simulink model "L1"  (R2023b)
settings: Solver=VariableStepAuto  StartTime=0.0  StopTime=10.0  RelTol=1e-3
values from neighbouring files (symbols this model uses):
  gravity = Airplane_data(52)    [Data_edit.m]
libraries: vrlib x6, dspmathops x4, matrix_library x1
settings Model: Creator=saifg  LastModifiedBy=saifg

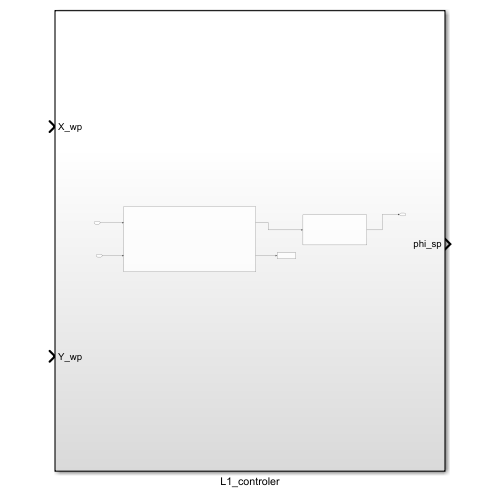
[thumbnail: Simulink's stored preview of the top-level diagram]
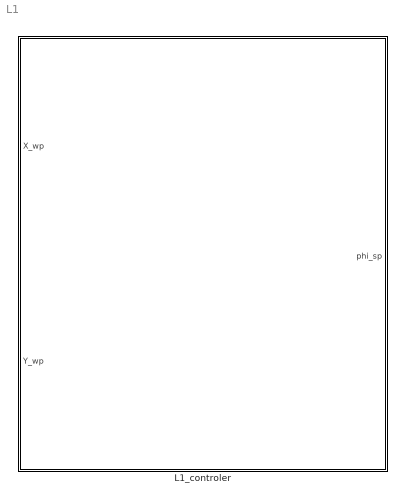
== system L1 ==
  L1_controler : Subsystem

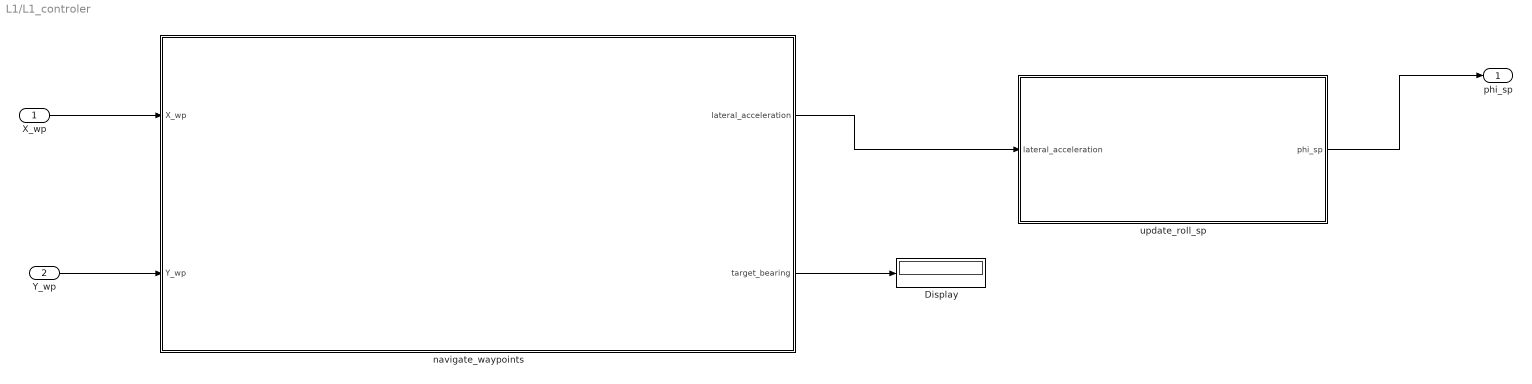
== system L1/L1_controler ==
  X_wp : Inport
  Y_wp : Inport  Port=2
  Display : Display
  navigate_waypoints : Subsystem
  update_roll_sp : Subsystem
  phi_sp : Outport
  wires:
  X_wp/1 -> navigate_waypoints/1(X_wp)
  Y_wp/1 -> navigate_waypoints/2(Y_wp)
  navigate_waypoints/2(target_bearing) -> Display/1
  navigate_waypoints/1(lateral_acceleration) -> update_roll_sp/1(lateral_acceleration)
  update_roll_sp/1(phi_sp) -> phi_sp/1

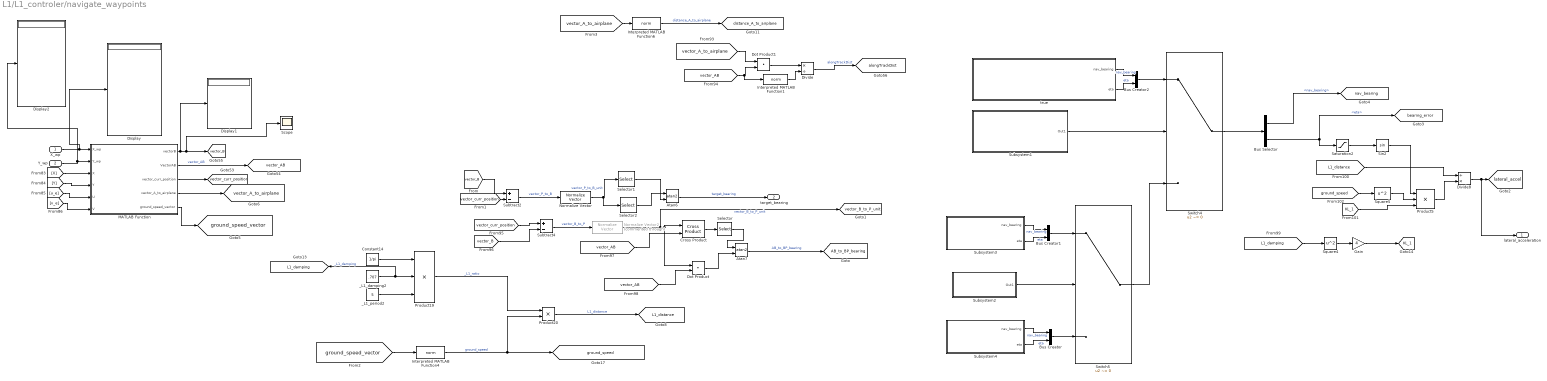
== system L1/L1_controler/navigate_waypoints ==
  X_wp : Inport
  Y_wp : Inport  Port=2
  Atan6 : Trigonometry  Operator=atan2
  Atan7 : Trigonometry  Operator=atan2
  Bus Creator : BusCreator  Inputs=2
  Bus Creator1 : BusCreator  Inputs=2
  Bus Creator2 : BusCreator  Inputs=2
  Bus Selector : BusSelector  OutputSignals=nav_bearing,eta
  Constant14 : Constant  Value=1/pi
  Cross Product : matrix_library/Cross Product
  Display : Display
  Display1 : Display
  Display2 : Display
  Divide : Product  Inputs=*/
  Divide8 : Product  Inputs=/*
  Dot Product : DotProduct  OutDataTypeStr=Inherit: Inherit via internal rule
  Dot Product1 : DotProduct  OutDataTypeStr=Inherit: Inherit via internal rule
  Gain : Gain  Gain=4
  Interpreted MATLAB Function1 : MATLABFcn  MATLABFcn=norm
  Interpreted MATLAB Function4 : MATLABFcn  MATLABFcn=norm
  Interpreted MATLAB Function6 : MATLABFcn  MATLABFcn=norm
  MATLAB Function : MATLAB Function  TreatAsAtomicUnit=on
  Normalize Vector : vrlib/Utilities/Normalize Vector  maxzero=0
  Normalize Vector2 : vrlib/Utilities/Normalize Vector  Commented=through  maxzero=0
  Product19 : Product  Inputs=3
  Product20 : Product
  Product5 : Product  Inputs=3
  Saturation2 : Saturate  UpperLimit=pi/2  LowerLimit=-pi/2
  Scope : Scope
  Selector : Selector  InputPortWidth=3  IndexOptions=Index vector (dialog)  Indices=3  OutputSizes=1
  Selector1 : Selector  InputPortWidth=3  IndexOptions=Index vector (dialog)  Indices=1  OutputSizes=1
  Selector2 : Selector  InputPortWidth=3  IndexOptions=Index vector (dialog)  Indices=2  OutputSizes=1
  Sin2 : Trigonometry
  Square4 : Math  Operator=square
  Square5 : Math  Operator=square
  Subsystem1 : Subsystem
  Subsystem2 : Subsystem
  Subsystem3 : Subsystem
  Subsystem4 : Subsystem
  Subtract2 : Sum  Inputs=+-
  Subtract4 : Sum  Inputs=+-
  Switch4 : Switch  Criteria=u2 ~= 0  SaturateOnIntegerOverflow=off  InputSameDT=off
  Switch5 : Switch  Criteria=u2 ~= 0  SaturateOnIntegerOverflow=off  InputSameDT=off
  _L1_damping2 : Constant  Value=.707
  _L1_period2 : Constant  Value=5
  true : Subsystem
  lateral_acceleration : Outport
  target_bearing : Outport  Port=2
  tag scope: AB_to_BP_bearing=global, KL_1=global, L1_damping=global, L1_distance=global, alongTrackDist=global, bearing_error=global, distance_A_to_airplane=global, ground_speed=global, ground_speed_vector=global, lateral_accel=global, nav_bearing=global, vector_AB=global, vector_A_to_airplane=global, vector_B=global, vector_B_to_P_unit=global, vector_curr_position=global
  wires:
  Dot Product/1 -> Atan7/2
  Divide/1 -> [alongTrackDist]  "alongTrackDist"
  Product19/1 -> Product20/1  "_L1_ratio"
  [ground_speed] -> Square5/1
  Sin2/1 -> Product5/1
  Interpreted MATLAB Function4/1 -> Product20/2, [ground_speed]  "ground_speed"
  MATLAB Function/2(VectorAB) -> [vector_AB]  "vector_AB"
  Normalize Vector/1 -> Selector2/1, Selector1/1  "vector_P_to_B_unit"
  Product20/1 -> [L1_distance]  "L1_distance"
  Y_wp/1 -> Display2/1, MATLAB Function/2(Y_wp)
  Atan7/1 -> [AB_to_BP_bearing]  "AB_to_BP_bearing"
  [L1_damping] -> Square4/1
  Constant14/1 -> Product19/1
  Subsystem1/1(Out1) -> Switch4/2
  Subtract2/1 -> Normalize Vector/1  "vector_P_to_B"
  [vector_A_to_airplane] -> Dot Product1/1
  X_wp/1 -> MATLAB Function/1(X_wp), Display/1
  [X] -> MATLAB Function/3(X)
  Divide8/1 -> lateral_acceleration/1, [lateral_accel]
  [Y] -> MATLAB Function/4(Y)
  Normalize Vector2/1 -> Dot Product/1, Cross Product/1, [vector_B_to_P_unit]  "vector_B_to_P_unit"
  Bus Creator2/1 -> Switch4/1
  [vector_B] -> Subtract4/2
  Subtract4/1 -> Normalize Vector2/1  "vector_B_to_P"
  [vector_curr_position] -> Subtract4/1
  [vector_AB] -> Interpreted MATLAB Function1/1, Dot Product1/2
  _L1_period2/1 -> Product19/3
  Bus Selector/1 -> [nav_bearing]  "<nav_bearing>"
  true/2(eta) -> Bus Creator2/2  "eta"
  _L1_damping2/1 -> [L1_damping], Product19/2  "_L1_damping"
  Bus Selector/2 -> Saturation2/1, [bearing_error]  "<eta>"
  Interpreted MATLAB Function6/1 -> [distance_A_to_airplane]  "distance_A_to_airplane"
  Switch5/1 -> Switch4/3
  Switch4/1 -> Bus Selector/1
  true/1(nav_bearing) -> Bus Creator2/1  "nav_bearing"
  Square4/1 -> Gain/1
  [L1_distance] -> Divide8/1
  Subsystem4/1(nav_bearing) -> Bus Creator/1  "nav_bearing"
  Subsystem4/2(eta) -> Bus Creator/2  "eta"
  Subsystem3/1(nav_bearing) -> Bus Creator1/1  "nav_bearing"
  Subsystem3/2(eta) -> Bus Creator1/2  "eta"
  Subsystem2/1(Out1) -> Switch5/2
  Saturation2/1 -> Sin2/1
  Product5/1 -> Divide8/2
  Atan6/1 -> target_bearing/1  "target_bearing"
  Gain/1 -> [KL_1]
  Square5/1 -> Product5/2
  [KL_1] -> Product5/3
  Bus Creator/1 -> Switch5/3
  Bus Creator1/1 -> Switch5/1
  [vector_AB] -> Dot Product/2
  Selector/1 -> Atan7/1
  Dot Product1/1 -> Divide/1
  Interpreted MATLAB Function1/1 -> Divide/2
  [vector_B] -> Subtract2/1
  [vector_curr_position] -> Subtract2/2
  MATLAB Function/1(vectorB) -> Display1/1, Scope/1, [vector_B]
  [vector_AB] -> Cross Product/2
  [u_e] -> MATLAB Function/5(U)
  [v_e] -> MATLAB Function/6(V)
  MATLAB Function/5(ground_speed_vector) -> [ground_speed_vector]
  [ground_speed_vector] -> Interpreted MATLAB Function4/1
  MATLAB Function/3(vector_curr_position) -> [vector_curr_position]
  MATLAB Function/4(vector_A_to_airplane) -> [vector_A_to_airplane]
  [vector_A_to_airplane] -> Interpreted MATLAB Function6/1
  Selector2/1 -> Atan6/1
  Selector1/1 -> Atan6/2
  Cross Product/1 -> Selector/1

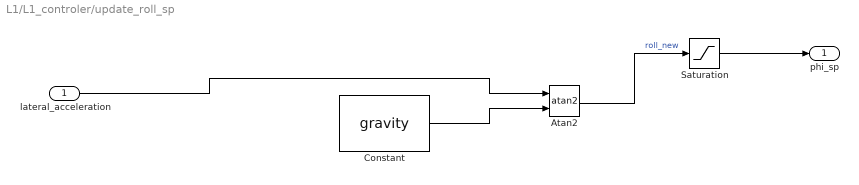
== system L1/L1_controler/update_roll_sp ==
  lateral_acceleration : Inport
  Atan2 : Trigonometry  Operator=atan2
  Constant : Constant  Value=gravity
  Saturation : Saturate  UpperLimit=deg2rad(70)  LowerLimit=-deg2rad(70)
  phi_sp : Outport
  wires:
  Saturation/1 -> phi_sp/1
  Constant/1 -> Atan2/2
  Atan2/1 -> Saturation/1  "roll_new"
  lateral_acceleration/1 -> Atan2/1

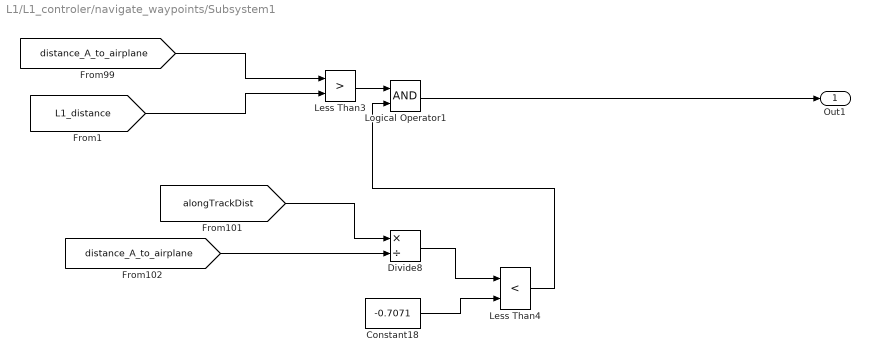
== system L1/L1_controler/navigate_waypoints/Subsystem1 ==
  Constant18 : Constant  Value=-0.7071
  Divide8 : Product  Inputs=*/
  Less Than3 : RelationalOperator  Operator=>  OutDataTypeStr=boolean  RndMeth=Simplest  InputSameDT=off
  Less Than4 : RelationalOperator  Operator=<  OutDataTypeStr=boolean  RndMeth=Simplest  InputSameDT=off
  Logical Operator1 : Logic  AllPortsSameDT=off  OutDataTypeStr=boolean
  Out1 : Outport
  wires:
  Less Than3/1 -> Logical Operator1/1
  Less Than4/1 -> Logical Operator1/2
  [distance_A_to_airplane] -> Less Than3/1
  Divide8/1 -> Less Than4/1
  Constant18/1 -> Less Than4/2
  [alongTrackDist] -> Divide8/1
  [L1_distance] -> Less Than3/2
  [distance_A_to_airplane] -> Divide8/2
  Logical Operator1/1 -> Out1/1

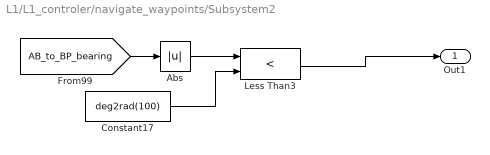
== system L1/L1_controler/navigate_waypoints/Subsystem2 ==
  Abs : Abs  SaturateOnIntegerOverflow=off
  Constant17 : Constant  Value=deg2rad(100)
  Less Than3 : RelationalOperator  Operator=<  OutDataTypeStr=boolean  RndMeth=Simplest  InputSameDT=off
  Out1 : Outport
  wires:
  Constant17/1 -> Less Than3/2
  [AB_to_BP_bearing] -> Abs/1
  Abs/1 -> Less Than3/1
  Less Than3/1 -> Out1/1

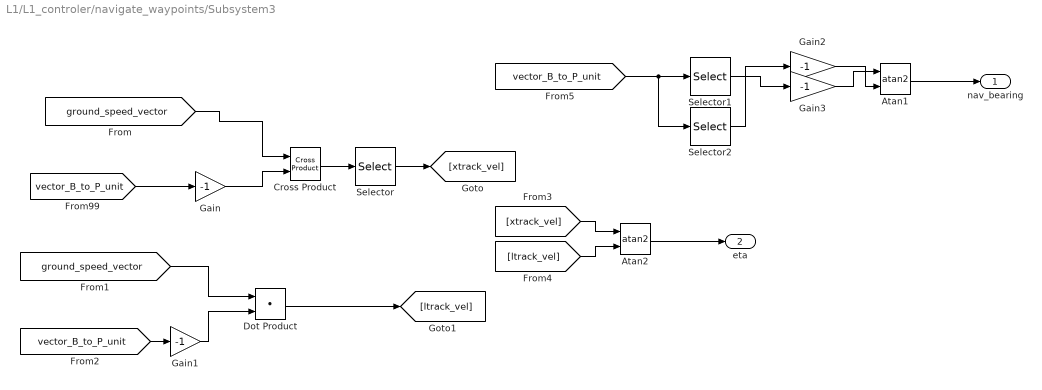
== system L1/L1_controler/navigate_waypoints/Subsystem3 ==
  Atan1 : Trigonometry  Operator=atan2
  Atan2 : Trigonometry  Operator=atan2
  Cross Product : vrlib/Utilities/Cross Product
  Dot Product : DotProduct  OutDataTypeStr=Inherit: Inherit via internal rule
  Gain{,1..3} (4 alike) : Gain  Gain=-1
  Selector : Selector  InputPortWidth=3  IndexOptions=Index vector (dialog)  Indices=3  OutputSizes=1
  Selector1 : Selector  InputPortWidth=3  IndexOptions=Index vector (dialog)  Indices=1  OutputSizes=1
  Selector2 : Selector  InputPortWidth=3  IndexOptions=Index vector (dialog)  Indices=2  OutputSizes=1
  nav_bearing : Outport
  eta : Outport  Port=2
  wires:
  [vector_B_to_P_unit] -> Gain/1
  Dot Product/1 -> [ltrack_vel]
  Gain1/1 -> Dot Product/2
  [vector_B_to_P_unit] -> Gain1/1
  [ground_speed_vector] -> Dot Product/1
  [xtrack_vel] -> Atan2/1
  [ltrack_vel] -> Atan2/2
  Atan2/1 -> eta/1
  Gain3/1 -> Atan1/1
  Gain2/1 -> Atan1/2
  Atan1/1 -> nav_bearing/1
  Gain/1 -> Cross Product/2
  [ground_speed_vector] -> Cross Product/1
  Cross Product/1 -> Selector/1
  Selector/1 -> [xtrack_vel]
  [vector_B_to_P_unit] -> Selector2/1, Selector1/1
  Selector1/1 -> Gain3/1
  Selector2/1 -> Gain2/1

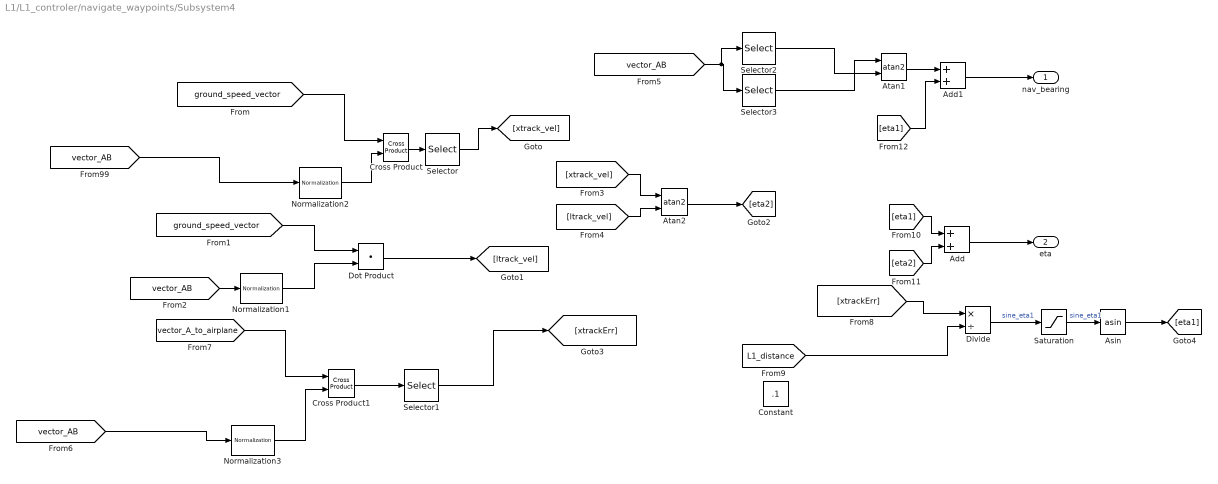
== system L1/L1_controler/navigate_waypoints/Subsystem4 ==
  Add : Sum
  Add1 : Sum
  Asin : Trigonometry  Operator=asin
  Atan1 : Trigonometry  Operator=atan2
  Atan2 : Trigonometry  Operator=atan2
  Constant : Constant  Value=.1
  Cross Product : vrlib/Utilities/Cross Product
  Cross Product1 : vrlib/Utilities/Cross Product
  Divide : Product  Inputs=*/
  Dot Product : DotProduct  OutDataTypeStr=Inherit: Inherit via internal rule
  Normalization1 : dspmathops/Normalization  NormType=2-norm  Bias=1e-10  NormOver=Each column  Dimension=1  roundingMode=Floor  overflowMode=off  accumDataTypeStr=Inherit: Same as product output  accumLastDataTypeStr=Inherit: Same as product output  outputDataTypeStr=Inherit: Same as product output  outputMin=[]  outputMax=[]  outputLastDataTypeStr=Inherit: Same as product output
  Normalization2 : dspmathops/Normalization  NormType=2-norm  Bias=1e-10  NormOver=Each column  Dimension=1  roundingMode=Floor  overflowMode=off  accumDataTypeStr=Inherit: Same as product output  accumLastDataTypeStr=Inherit: Same as product output  outputDataTypeStr=Inherit: Same as product output  outputMin=[]  outputMax=[]  outputLastDataTypeStr=Inherit: Same as product output
  Normalization3 : dspmathops/Normalization  NormType=2-norm  Bias=1e-10  NormOver=Each column  Dimension=1  roundingMode=Floor  overflowMode=off  accumDataTypeStr=Inherit: Same as product output  accumLastDataTypeStr=Inherit: Same as product output  outputDataTypeStr=Inherit: Same as product output  outputMin=[]  outputMax=[]  outputLastDataTypeStr=Inherit: Same as product output
  Saturation : Saturate  UpperLimit=sin(pi/4)  LowerLimit=-sin(pi/4)
  Selector : Selector  InputPortWidth=3  IndexOptions=Index vector (dialog)  Indices=[3]  OutputSizes=1
  Selector1 : Selector  InputPortWidth=3  IndexOptions=Index vector (dialog)  Indices=[3]  OutputSizes=1
  Selector2 : Selector  InputPortWidth=3  IndexOptions=Index vector (dialog)  Indices=1  OutputSizes=1
  Selector3 : Selector  InputPortWidth=3  IndexOptions=Index vector (dialog)  Indices=2  OutputSizes=1
  nav_bearing : Outport
  eta : Outport  Port=2
  wires:
  [ltrack_vel] -> Atan2/2
  [xtrack_vel] -> Atan2/1
  [ground_speed_vector] -> Dot Product/1
  [vector_AB] -> Normalization1/1
  Dot Product/1 -> [ltrack_vel]
  Atan2/1 -> [eta2]
  [xtrackErr] -> Divide/1
  [L1_distance] -> Divide/2
  Divide/1 -> Saturation/1  "sine_eta1"
  Saturation/1 -> Asin/1  "sine_eta1"
  Asin/1 -> [eta1]
  [eta1] -> Add/1
  [eta2] -> Add/2
  Add/1 -> eta/1
  Atan1/1 -> Add1/1
  [eta1] -> Add1/2
  Add1/1 -> nav_bearing/1
  [vector_AB] -> Normalization2/1
  [ground_speed_vector] -> Cross Product/1
  Cross Product/1 -> Selector/1
  Selector/1 -> [xtrack_vel]
  [vector_A_to_airplane] -> Cross Product1/1
  [vector_AB] -> Normalization3/1
  Cross Product1/1 -> Selector1/1
  Selector1/1 -> [xtrackErr]
  Normalization1/1 -> Dot Product/2
  Normalization2/1 -> Cross Product/2
  Normalization3/1 -> Cross Product1/2
  [vector_AB] -> Selector2/1, Selector3/1
  Selector3/1 -> Atan1/1
  Selector2/1 -> Atan1/2

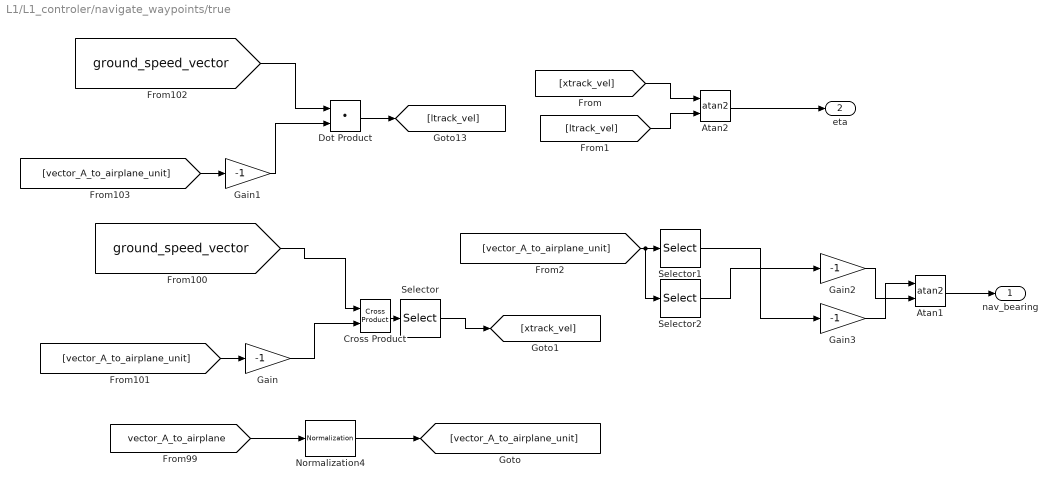
== system L1/L1_controler/navigate_waypoints/true ==
  Atan1 : Trigonometry  Operator=atan2
  Atan2 : Trigonometry  Operator=atan2
  Cross Product : vrlib/Utilities/Cross Product
  Dot Product : DotProduct  OutDataTypeStr=Inherit: Inherit via internal rule
  Gain{,1..3} (4 alike) : Gain  Gain=-1
  Normalization4 : dspmathops/Normalization  NormType=2-norm  Bias=1e-10  NormOver=Each column  Dimension=1  roundingMode=Floor  overflowMode=off  accumDataTypeStr=Inherit: Same as product output  accumLastDataTypeStr=Inherit: Same as product output  outputDataTypeStr=Inherit: Same as product output  outputMin=[]  outputMax=[]  outputLastDataTypeStr=Inherit: Same as product output
  Selector : Selector  InputPortWidth=3  IndexOptions=Index vector (dialog)  Indices=3  OutputSizes=1
  Selector1 : Selector  InputPortWidth=3  IndexOptions=Index vector (dialog)  Indices=1  OutputSizes=1
  Selector2 : Selector  InputPortWidth=3  IndexOptions=Index vector (dialog)  Indices=2  OutputSizes=1
  nav_bearing : Outport
  eta : Outport  Port=2
  wires:
  [vector_A_to_airplane_unit] -> Gain1/1
  Gain1/1 -> Dot Product/2
  [vector_A_to_airplane] -> Normalization4/1
  [vector_A_to_airplane_unit] -> Gain/1
  [ground_speed_vector] -> Dot Product/1
  Normalization4/1 -> [vector_A_to_airplane_unit]
  Dot Product/1 -> [ltrack_vel]
  [ltrack_vel] -> Atan2/2
  [xtrack_vel] -> Atan2/1
  Atan2/1 -> eta/1
  [vector_A_to_airplane_unit] -> Selector2/1, Selector1/1
  Selector2/1 -> Gain2/1
  Selector1/1 -> Gain3/1
  Gain3/1 -> Atan1/1
  Gain2/1 -> Atan1/2
  Atan1/1 -> nav_bearing/1
  [ground_speed_vector] -> Cross Product/1
  Gain/1 -> Cross Product/2
  Cross Product/1 -> Selector/1
  Selector/1 -> [xtrack_vel]

== matlab function L1/L1_controler/navigate_waypoints/MATLAB Function ==
  data: X_wp input; vectorB output; Y_wp input; VectorAB output; vector_curr_position output; X input; Y input; vector_A_to_airplane output; U input; V input; ground_speed_vector output
function [vectorB,VectorAB,vector_curr_position,vector_A_to_airplane,ground_speed_vector]= fcn(X_wp, Y_wp, X,Y,U,V)

n=length(X_wp);
vector_curr_position=[X,Y,0];
ground_speed_vector=[U,V,0];
 for i=2:n
    vectorB=[X_wp(i),Y_wp(i),0];
    VectorAB=vectorB-[X_wp(i-1),Y_wp(i-1),0];
    vector_A_to_airplane=vector_curr_position-[X_wp(i-1),Y_wp(i-1),0];
end
